simulink model "six_phase_Rectifier"  (R2017b)
settings: Solver=VariableStepAuto  StartTime=0.0  StopTime=0.06  MaxStep=1e-4  RelTol=1e-3
libraries: powerlib x19
settings Model: Creator=sepykian  LastModifiedBy=sepykian

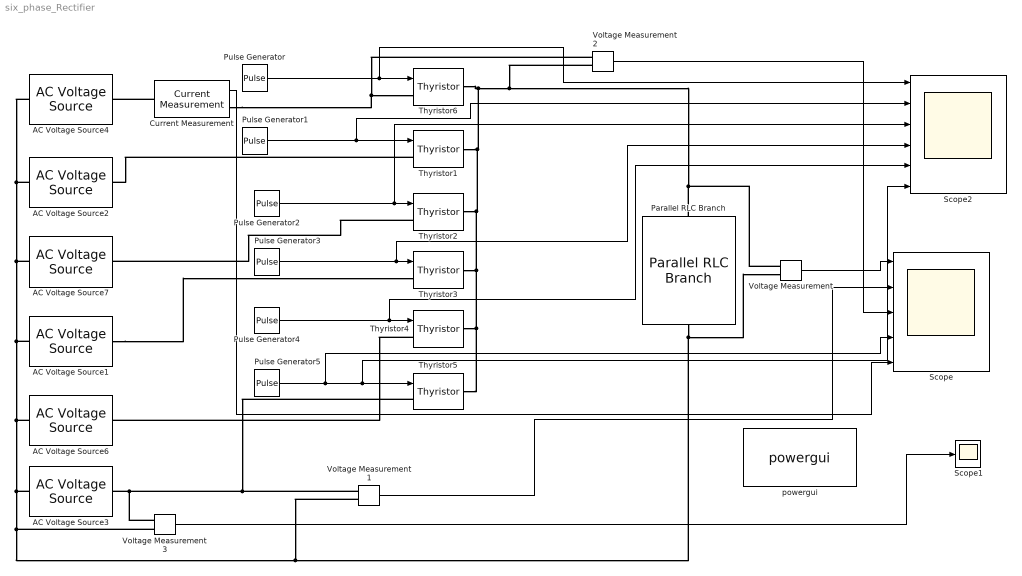
== system six_phase_Rectifier ==
  AC Voltage Source1 : powerlib/Electrical Sources/AC Voltage Source  Amplitude=100  Phase=-180  Frequency=50  SampleTime=0  Measurements=None  BusType=swing  Pref=10e3  Qref=0  Qmin=-inf  Qmax=+inf
  AC Voltage Source2 : powerlib/Electrical Sources/AC Voltage Source  Amplitude=100  Phase=-60  Frequency=50  SampleTime=0  Measurements=None  BusType=swing  Pref=10e3  Qref=0  Qmin=-inf  Qmax=+inf
  AC Voltage Source3 : powerlib/Electrical Sources/AC Voltage Source  Amplitude=100  Phase=-300  Frequency=50  SampleTime=0  Measurements=None  BusType=swing  Pref=10e3  Qref=0  Qmin=-inf  Qmax=+inf
  AC Voltage Source4 : powerlib/Electrical Sources/AC Voltage Source  Amplitude=100  Phase=0  Frequency=50  SampleTime=0  Measurements=None  BusType=swing  Pref=10e3  Qref=0  Qmin=-inf  Qmax=+inf
  AC Voltage Source6 : powerlib/Electrical Sources/AC Voltage Source  Amplitude=100  Phase=-240  Frequency=50  SampleTime=0  Measurements=None  BusType=swing  Pref=10e3  Qref=0  Qmin=-inf  Qmax=+inf
  AC Voltage Source7 : powerlib/Electrical Sources/AC Voltage Source  Amplitude=100  Phase=-120  Frequency=50  SampleTime=0  Measurements=None  BusType=swing  Pref=10e3  Qref=0  Qmin=-inf  Qmax=+inf
  Current Measurement : powerlib/Measurements/Current Measurement  PhasorSimulation=off  OutputType=Complex  PSBequivalent=0
  Parallel RLC Branch : powerlib/Elements/Parallel RLC Branch  LConnTagsString=a  RConnTagsString=__new0  BranchType=R  Resistance=134  Inductance=1e-3  SetiL0=off  InitialCurrent=0  Capacitance=1e-6  Setx0=off  InitialVoltage=0  Measurements=None
  Pulse Generator : DiscretePulseGenerator  PulseType=Time based  Period=0.02  PulseWidth=50  PhaseDelay=(0.01/3)+(0.09/18)
  Pulse Generator1 : DiscretePulseGenerator  PulseType=Time based  Period=0.02  PulseWidth=50  PhaseDelay=(0.02/3)+(0.09/18)
  Pulse Generator2 : DiscretePulseGenerator  PulseType=Time based  Period=0.02  PulseWidth=50  PhaseDelay=(0.03/3)+(0.09/18)
  Pulse Generator3 : DiscretePulseGenerator  PulseType=Time based  Period=0.02  PulseWidth=50  PhaseDelay=(0.04/3)+(0.09/18)
  Pulse Generator4 : DiscretePulseGenerator  PulseType=Time based  Period=0.02  PulseWidth=50  PhaseDelay=(0.05/3)+(0.09/18)
  Pulse Generator5 : DiscretePulseGenerator  PulseType=Time based  Period=0.02  PulseWidth=50  PhaseDelay=(0.09/18)
  Scope : Scope  NumInputPorts=5
  Scope1 : Scope
  Scope2 : Scope  NumInputPorts=6
  Thyristor{1..6} (6 alike) : powerlib/Power Electronics/Thyristor  Ron=0.001  Lon=0  Vf=0.8  IC=0  Rs=500  Cs=250e-9  Measurements=off
  Voltage Measurement{,1..3} (4 alike) : powerlib/Measurements/Voltage Measurement  PhasorSimulation=off  OutputType=Complex  PSBequivalent=0
  powergui : powerlib/powergui  Priority=1  SimulationMode=Continuous  SampleTime=50e-6  frequency=60  Iterations=50  frequencyindice=50  Pbase=100e6  ErrMax=1e-4  UnitsV=kV  UnitsW=MW  buscounter=0  FunctionMessages=off  echomessages=off  EnableUseOfTLC=off  CurrentSourceSwitches=off  DisableSnubberDevices=off  DisableRonSwitches=off  DisableVfSwitches=off  DisplayEquations=off  SolverType=Tustin/Backward Euler (TBE)  Interpol=off  ExternalGateDelay=off  methode=off  Ts=100  x0status=blocks  SPID=on  SwTol=0  HookPort=off  RestoreLinks=warning  ResistiveCurrentMeasurement=off  Frange=[0:2:500]  Ylog=off  Xlog=on  ShowGrid=off  save=off  variable=ZData  structure=0  ZoomFFT=off  StartTime=0.0  cycles=1  DisplayStyle=1  fundamental=60  FreqAxis=off  MaxFrequency=1000  frequencyindicesteady=1  RmsSteady=1  display=off
  wires:
  Pulse Generator3/1 -> Scope2/4, Thyristor3/1
  Pulse Generator/1 -> Scope2/1, Thyristor6/1
  Pulse Generator2/1 -> Scope2/3, Thyristor2/1
  Voltage Measurement/1 -> Scope/1
  Pulse Generator5/1 -> Scope/4, Scope2/6, Thyristor5/1
  Pulse Generator4/1 -> Scope2/5, Thyristor4/1
  Pulse Generator1/1 -> Scope2/2, Thyristor1/1
  Voltage Measurement1/1 -> Scope/2
  Voltage Measurement2/1 -> Scope/3
  Current Measurement/1 -> Scope/5
  Voltage Measurement3/1 -> Scope1/1
  connections:
  AC Voltage Source4/LConn1 -- AC Voltage Source2/LConn1 -- AC Voltage Source7/LConn1 -- AC Voltage Source1/LConn1 -- AC Voltage Source3/LConn1 -- Voltage Measurement3/LConn2 -- Voltage Measurement1/LConn2 -- Voltage Measurement/LConn2 -- Parallel RLC Branch/RConn1 -- AC Voltage Source6/LConn1
  Thyristor2/LConn1 -- AC Voltage Source7/RConn1
  Thyristor1/LConn1 -- AC Voltage Source2/RConn1
  Voltage Measurement/LConn1 -- Voltage Measurement2/LConn2 -- Thyristor5/RConn1 -- Thyristor4/RConn1 -- Thyristor3/RConn1 -- Thyristor2/RConn1 -- Thyristor1/RConn1 -- Thyristor6/RConn1 -- Parallel RLC Branch/LConn1
  Voltage Measurement2/LConn1 -- Current Measurement/RConn1 -- Thyristor6/LConn1
  Thyristor4/LConn1 -- AC Voltage Source6/RConn1
  Thyristor5/LConn1 -- Voltage Measurement3/LConn1 -- AC Voltage Source3/RConn1 -- Voltage Measurement1/LConn1
  AC Voltage Source1/RConn1 -- Thyristor3/LConn1
  Current Measurement/LConn1 -- AC Voltage Source4/RConn1
